simulink model "PI_park_filter_linearLoad"  (R2017b)
settings: Solver=ode23tb  StartTime=0.0  StopTime=.6  MaxStep=1e-4  RelTol=1e-3
undefined symbols (not defined in the file): D1, Delta
libraries: powerlib x42, powerlib_extras x9, powerlib_meascontrol x3, sdolib x1, peSinusoidalMeasurement x1
settings Model: Creator=HP  LastModifiedBy=HP

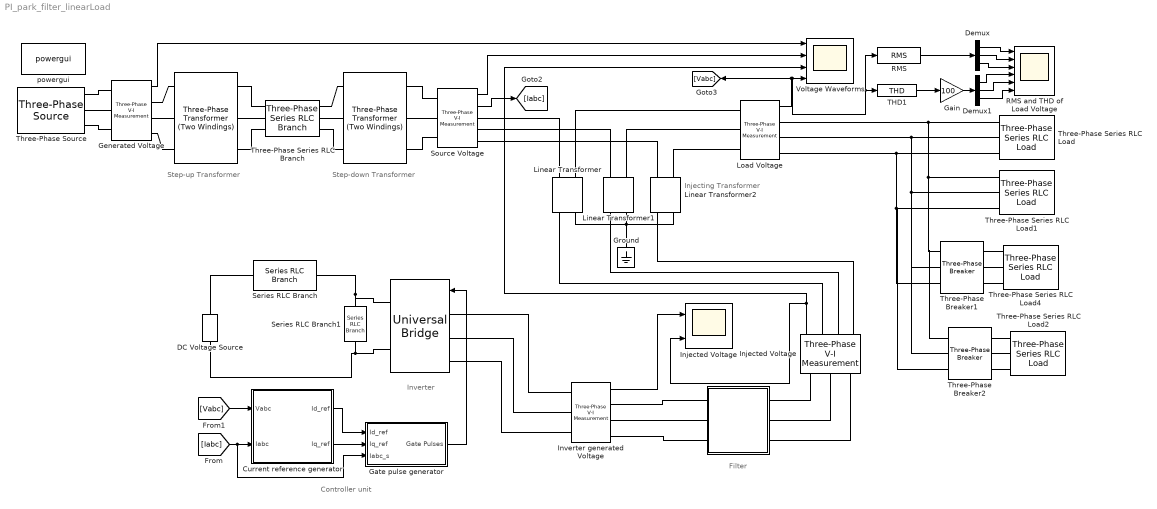
== system PI_park_filter_linearLoad ==
  note: Step-up Transformer
  note: Controller unit
  note: Injecting Transformer
  note: Step-down Transformer
  note: Inverter
  note: Filter
  " " : powerlib/Elements/Three-Phase Transformer (Two Windings)  Winding1Connection=Yg  Winding2Connection=Delta (D1)  CoreType=Three single-phase transformers  SetSaturation=off  Hysteresis=off  DataFile='hysteresis'  SetInitialFlux=off  Measurements=None  UNITS=pu  NominalPower=[ 70e6 , 50 ]  Winding1=[ 13e3 , 0.002 , 0.08 ]  Winding2=[ 115e3 , 0.002 , 0.08 ]  Rm=500  Lm=1400  L0=0.5  Saturation=[ 0,0 ; 0.0024,1.2 ; 1.0,1.52 ]  InitialFluxes=[ 0.8 , -0.8 , 0.7 ]  MoreParameters=off  BreakLoop=off  DataType=off  TransfoNumber=1
  " " : Subsystem
  "      " : powerlib/Elements/Three-Phase Transformer (Two Windings)  Winding1Connection=Delta (D1)  Winding2Connection=Yg  CoreType=Three single-phase transformers  SetSaturation=off  Hysteresis=off  DataFile='hysteresis'  SetInitialFlux=off  Measurements=None  UNITS=pu  NominalPower=[ 70e6 , 50 ]  Winding1=[ 115e3 , 0.002 , 0.08 ]  Winding2=[ 11e3 , 0.002 , 0.08 ]  Rm=500  Lm=800  L0=0.5  Saturation=[ 0,0 ; 0.0024,1.2 ; 1.0,1.52 ]  InitialFluxes=[ 0.8 , -0.8 , 0.7 ]  MoreParameters=off  BreakLoop=off  DataType=off  TransfoNumber=1
  "                                 " : powerlib/Power Electronics/Universal Bridge  Arms=3  SnubberResistance=1e5  SnubberCapacitance=inf  Device=IGBT / Diodes  Ron=1  Lon=0  ForwardVoltages="[  0  0  ]"  ForwardVoltage=0  GTOparameters=[ 10e-6 , 20e-6 ]  IGBTparameters=[ 1e-6 , 2e-6 ]  Measurements=None  Measurements_2=None  converterType=Rectifier
  Current reference generator : Subsystem
  "DC Voltage Source " : powerlib/Electrical Sources/DC Voltage Source  Amplitude=400  Measurements=None
  Demux : Demux  Outputs=3
  Demux1 : Demux  Outputs=3
  Gain : Gain  Gain=100
  "Gate pulse generator " : Subsystem
  Generated Voltage : powerlib/Measurements/Three-Phase V-I Measurement  VoltageMeasurement=phase-to-ground  SetLabelV=off  LabelV=Vabc  Vpu=off  VpuLL=off  CurrentMeasurement=no  SetLabelI=off  LabelI=Iabc  Ipu=off  Pbase=100e6  Vbase=11e3  OutputType=Complex  PhasorSimulation=off  PSBequivalent=0
  Ground : powerlib/Elements/Ground  LConnTagsString=a
  Injected Voltage : powerlib/Measurements/Three-Phase V-I Measurement  VoltageMeasurement=phase-to-ground  SetLabelV=off  LabelV=Vabc  Vpu=off  VpuLL=off  CurrentMeasurement=no  SetLabelI=off  LabelI=Iabc  Ipu=off  Pbase=100e6  Vbase=11e3  OutputType=Complex  PhasorSimulation=off  PSBequivalent=0
  "Injected Voltage " : Scope  NumInputPorts=2
  Inverter generated Voltage : powerlib/Measurements/Three-Phase V-I Measurement  VoltageMeasurement=phase-to-ground  SetLabelV=off  LabelV=Vabc  Vpu=off  VpuLL=off  CurrentMeasurement=no  SetLabelI=off  LabelI=Iabc  Ipu=off  Pbase=100e6  Vbase=11e3  OutputType=Complex  PhasorSimulation=off  PSBequivalent=0
  Linear Transformer : powerlib/Elements/Linear Transformer  UNITS=pu  NominalPower=[ 250e6 50 ]  winding1="[ 11e3  0.002  0.08 ]"  winding2="[ 22e3  0.002  0.08 ]"  ThreeWindings=off  winding3=[ 315e3 0.002 0.08 ]  RmLm=[ 500 750 ]  Measurements=None  DataType=off
  Linear Transformer1 : powerlib/Elements/Linear Transformer  UNITS=pu  NominalPower=[ 250e6 50 ]  winding1="[ 11e3  0.002  0.08 ]"  winding2="[ 22e3  0.002  0.08 ]"  ThreeWindings=off  winding3=[ 315e3 0.002 0.08 ]  RmLm=[ 500 750 ]  Measurements=None  DataType=off
  Linear Transformer2 : powerlib/Elements/Linear Transformer  UNITS=pu  NominalPower=[ 250e6 50 ]  winding1="[ 11e3  0.002  0.08 ]"  winding2="[ 22e3  0.002  0.08 ]"  ThreeWindings=off  winding3=[ 315e3 0.002 0.08 ]  RmLm=[ 500 750 ]  Measurements=None  DataType=off
  Load Voltage : powerlib/Measurements/Three-Phase V-I Measurement  VoltageMeasurement=phase-to-ground  SetLabelV=off  LabelV=Vabc  Vpu=off  VpuLL=off  CurrentMeasurement=no  SetLabelI=off  LabelI=Iabc  Ipu=off  Pbase=100e6  Vbase=11e3  OutputType=Complex  PhasorSimulation=off  PSBequivalent=0
  RMS : powerlib_meascontrol/Measurements/RMS  TrueRMS=on  Freq=50  RMSInit=120  Ts=0
  RMS and THD of Load Voltage : Scope  NumInputPorts=6
  Series RLC Branch : powerlib/Elements/Series RLC Branch  LConnTagsString=__new0  RConnTagsString=__new0  BranchType=R  Resistance=20  Inductance=0  SetiL0=off  InitialCurrent=0  Capacitance=0  Setx0=off  InitialVoltage=0  Measurements=None
  Series RLC Branch1 : powerlib/Elements/Series RLC Branch  LConnTagsString=__new0  RConnTagsString=__new0  BranchType=C  Resistance=10  Inductance=0  SetiL0=off  InitialCurrent=0  Capacitance=1e-3  Setx0=off  InitialVoltage=0  Measurements=None
  Source Voltage : powerlib/Measurements/Three-Phase V-I Measurement  VoltageMeasurement=phase-to-ground  SetLabelV=off  LabelV=Vabc  Vpu=off  VpuLL=off  CurrentMeasurement=yes  SetLabelI=off  LabelI=Iabc  Ipu=off  Pbase=100e6  Vbase=11e3  OutputType=Complex  PhasorSimulation=off  PSBequivalent=0
  THD1 : powerlib_meascontrol/Measurements/THD  Freq=50  Ts=0
  Three-Phase Series RLC Branch : powerlib/Elements/Three-Phase Series RLC Branch  LConnTagsString=A|B|C  RConnTagsString=A|B|C  BranchType=RL  Resistance=.1  Inductance=.5e-3  Capacitance=1e-6  Measurements=None
  Three-Phase Series RLC Load : powerlib/Elements/Three-Phase Series RLC Load  LConnTagsString=A|B|C  Configuration=Y (grounded)  NominalVoltage=11000  Vabc=[1e3 1e3 1e3]  Vabcp=[1e3 1e3 1e3]  NominalFrequency=50  UnbalancedPower=off  ActivePower=20e3  InductivePower=60e3  CapacitivePower=0  Pabc=[10e3 9e3 11e3]  QLabc=[100 90 110]  QCabc=[100 90 110]  Pabcp=[10e3 9e3 11e3]  QLabcp=[100 90 110]  QCabcp=[100 90 110]  Measurements=None  LoadType=constant Z
  Three-Phase Series RLC Load1 : powerlib/Elements/Three-Phase Series RLC Load  LConnTagsString=A|B|C  Configuration=Y (grounded)  NominalVoltage=11000  Vabc=[1e3 1e3 1e3]  Vabcp=[1e3 1e3 1e3]  NominalFrequency=50  UnbalancedPower=off  ActivePower=20e3  InductivePower=60e3  CapacitivePower=0  Pabc=[10e3 9e3 11e3]  QLabc=[100 90 110]  QCabc=[100 90 110]  Pabcp=[10e3 9e3 11e3]  QLabcp=[100 90 110]  QCabcp=[100 90 110]  Measurements=None  LoadType=constant Z
  Three-Phase Series RLC Load2 : powerlib/Elements/Three-Phase Series RLC Load  LConnTagsString=A|B|C  Configuration=Y (grounded)  NominalVoltage=11000  Vabc=[1e3 1e3 1e3]  Vabcp=[1e3 1e3 1e3]  NominalFrequency=50  UnbalancedPower=off  ActivePower=300e3  InductivePower=0  CapacitivePower=0  Pabc=[10e3 9e3 11e3]  QLabc=[100 90 110]  QCabc=[100 90 110]  Pabcp=[10e3 9e3 11e3]  QLabcp=[100 90 110]  QCabcp=[100 90 110]  Measurements=None  LoadType=constant Z
  Three-Phase Series RLC Load4 : powerlib/Elements/Three-Phase Series RLC Load  LConnTagsString=A|B|C  Configuration=Y (grounded)  NominalVoltage=11000  Vabc=[1e3 1e3 1e3]  Vabcp=[1e3 1e3 1e3]  NominalFrequency=50  UnbalancedPower=off  ActivePower=350e3  InductivePower=0  CapacitivePower=0  Pabc=[10e3 9e3 11e3]  QLabc=[100 90 110]  QCabc=[100 90 110]  Pabcp=[10e3 9e3 11e3]  QLabcp=[100 90 110]  QCabcp=[100 90 110]  Measurements=None  LoadType=constant Z
  Three-Phase Breaker1 : powerlib/Elements/Three-Phase Breaker  InitialState=open  SwitchA=on  SwitchB=on  SwitchC=on  SwitchTimes="[10/50  ]"  External=off  BreakerResistance=0.01  SnubberResistance=1e6  SnubberCapacitance=inf  Measurements=None
  Three-Phase Breaker2 : powerlib/Elements/Three-Phase Breaker  InitialState=open  SwitchA=on  SwitchB=on  SwitchC=on  SwitchTimes="[20/50  ]"  External=off  BreakerResistance=0.01  SnubberResistance=1e6  SnubberCapacitance=inf  Measurements=None
  Three-Phase Source : powerlib/Electrical Sources/Three-Phase Source  InternalConnection=Yg  VoltagePhases=off  Voltage=13e3  PhaseAngle=0  Voltage_phases=[25e3 25e3 25e3]/sqrt(3)  PhaseAngles_phases=[0 -120 +120]  Frequency=50  NonIdealSource=on  SpecifyImpedance=off  Resistance=0.2929  Inductance=16.58e-3  ShortCircuitLevel=100e6  BaseVoltage=13e3  XRratio=7  BusType=swing  Pref=10e3  Qref=0  Prefabc=[10e3, 10e3, 10e3]  Qrefabc=[0, 0, 0]  Qmin=-inf  Qmax=inf
  "Voltage Waveforms " : Scope  NumInputPorts=4
  powergui : powerlib/powergui  Priority=1  SimulationMode=Discrete  SampleTime=50e-6  frequency=60  Iterations=50  frequencyindice=50  Pbase=100e6  ErrMax=1e-4  UnitsV=kV  UnitsW=MW  buscounter=0  FunctionMessages=off  echomessages=off  EnableUseOfTLC=off  CurrentSourceSwitches=off  DisableSnubberDevices=off  DisableRonSwitches=off  DisableVfSwitches=off  DisplayEquations=off  SolverType=Tustin/Backward Euler (TBE)  Interpol=off  ExternalGateDelay=off  methode=off  Ts=100  x0status=blocks  SPID=on  SwTol=0  HookPort=off  RestoreLinks=warning  ResistiveCurrentMeasurement=off  Frange=[0:2:500]  Ylog=off  Xlog=on  ShowGrid=off  save=off  variable=ZData  structure=WAVEFORMS_PI_PARK_Linear  ZoomFFT=off  StartTime=0.  cycles=30  DisplayStyle=1  fundamental=50  FreqAxis=off  MaxFrequency=1000  frequencyindicesteady=1  RmsSteady=1  display=off
  wires:
  [Vabc] -> Current reference generator/1(Vabc)
  [Iabc] -> "Gate pulse generator "/3(Iabc_s), Current reference generator/2(Iabc)
  Current reference generator/1(Id_ref) -> "Gate pulse generator "/1(Id_ref)
  Current reference generator/2(Iq_ref) -> "Gate pulse generator "/2(Iq_ref)
  "Gate pulse generator "/1("Gate Pulses ") -> "                                 "/1
  Source Voltage/2 -> [Iabc]
  Load Voltage/1 -> RMS/1, THD1/1, "Voltage Waveforms "/4, [Vabc]
  Generated Voltage/1 -> "Voltage Waveforms "/1
  Source Voltage/1 -> "Voltage Waveforms "/2
  Injected Voltage/1 -> "Injected Voltage "/2, "Voltage Waveforms "/3
  Inverter generated Voltage/1 -> "Injected Voltage "/1
  Demux/1 -> RMS and THD of Load Voltage/1
  Demux/2 -> RMS and THD of Load Voltage/2
  Demux/3 -> RMS and THD of Load Voltage/3
  Demux1/2 -> RMS and THD of Load Voltage/5
  Demux1/1 -> RMS and THD of Load Voltage/4
  Demux1/3 -> RMS and THD of Load Voltage/6
  THD1/1 -> Gain/1
  Gain/1 -> Demux1/1
  RMS/1 -> Demux/1
  connections:
  "DC Voltage Source "/RConn1 -- Series RLC Branch/LConn1
  Series RLC Branch1/LConn1 -- "                                 "/RConn1 -- Series RLC Branch/RConn1
  "DC Voltage Source "/LConn1 -- "                                 "/RConn2 -- Series RLC Branch1/RConn1
  Three-Phase Series RLC Load1/LConn3 -- Three-Phase Breaker2/LConn3 -- Three-Phase Breaker1/LConn3 -- Three-Phase Series RLC Load/LConn3 -- Load Voltage/RConn3
  Three-Phase Series RLC Load1/LConn1 -- Three-Phase Breaker2/LConn1 -- Three-Phase Breaker1/LConn1 -- Three-Phase Series RLC Load/LConn1 -- Load Voltage/RConn1
  Three-Phase Series RLC Load1/LConn2 -- Three-Phase Breaker2/LConn2 -- Three-Phase Breaker1/LConn2 -- Load Voltage/RConn2 -- Three-Phase Series RLC Load/LConn2
  Linear Transformer2/LConn1 -- Load Voltage/LConn3
  " "/LConn2 -- Generated Voltage/RConn2
  Three-Phase Series RLC Branch/LConn1 -- " "/RConn1
  Generated Voltage/RConn1 -- " "/LConn1
  "      "/RConn3 -- Source Voltage/LConn3
  Three-Phase Source/RConn3 -- Generated Voltage/LConn3
  " "/LConn3 -- Generated Voltage/RConn3
  Source Voltage/LConn1 -- "      "/RConn1
  Three-Phase Source/RConn1 -- Generated Voltage/LConn1
  Three-Phase Series RLC Branch/LConn2 -- " "/RConn2
  Generated Voltage/LConn2 -- Three-Phase Source/RConn2
  Linear Transformer/LConn1 -- Load Voltage/LConn1
  Source Voltage/RConn1 -- Linear Transformer/LConn2
  Load Voltage/LConn2 -- Linear Transformer1/LConn1
  Source Voltage/RConn3 -- Linear Transformer2/LConn2
  Source Voltage/LConn2 -- "      "/RConn2
  Three-Phase Series RLC Branch/RConn1 -- "      "/LConn1
  Three-Phase Series RLC Branch/RConn3 -- "      "/LConn3
  Three-Phase Series RLC Branch/RConn2 -- "      "/LConn2
  Three-Phase Series RLC Branch/LConn3 -- " "/RConn3
  Source Voltage/RConn2 -- Linear Transformer1/LConn2
  Linear Transformer/RConn1 -- Ground/LConn1 -- Linear Transformer1/RConn1 -- Linear Transformer2/RConn1
  Injected Voltage/RConn1 -- Linear Transformer/RConn2
  Injected Voltage/RConn2 -- Linear Transformer1/RConn2
  Injected Voltage/RConn3 -- Linear Transformer2/RConn2
  Inverter generated Voltage/LConn1 -- "                                 "/LConn1
  Inverter generated Voltage/LConn2 -- "                                 "/LConn2
  Inverter generated Voltage/LConn3 -- "                                 "/LConn3
  " "/RConn1 -- Injected Voltage/LConn1
  " "/RConn2 -- Injected Voltage/LConn2
  " "/RConn3 -- Injected Voltage/LConn3
  Inverter generated Voltage/RConn1 -- " "/LConn1
  Inverter generated Voltage/RConn2 -- " "/LConn2
  Inverter generated Voltage/RConn3 -- " "/LConn3
  Three-Phase Series RLC Load4/LConn3 -- Three-Phase Breaker1/RConn3
  Three-Phase Series RLC Load4/LConn2 -- Three-Phase Breaker1/RConn2
  Three-Phase Series RLC Load4/LConn1 -- Three-Phase Breaker1/RConn1
  Three-Phase Series RLC Load2/LConn1 -- Three-Phase Breaker2/RConn1
  Three-Phase Series RLC Load2/LConn2 -- Three-Phase Breaker2/RConn2
  Three-Phase Series RLC Load2/LConn3 -- Three-Phase Breaker2/RConn3

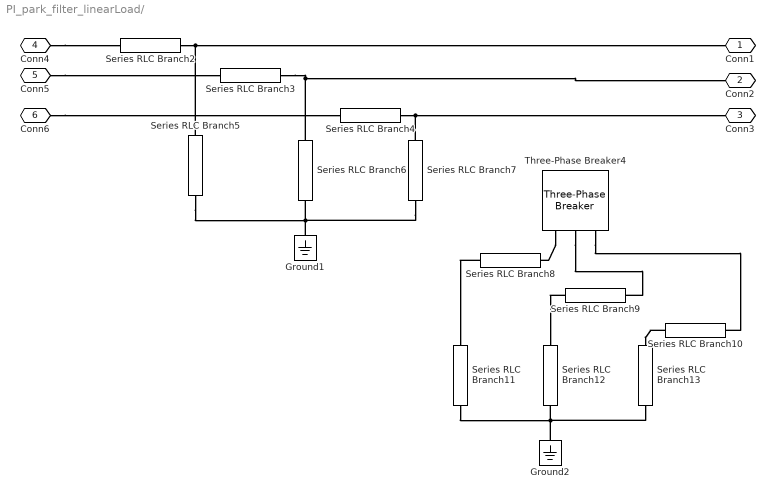
== system PI_park_filter_linearLoad/  ==
  Ground1 : powerlib/Elements/Ground  LConnTagsString=a
  Ground2 : powerlib/Elements/Ground  LConnTagsString=a
  Series RLC Branch10 : powerlib/Elements/Series RLC Branch  LConnTagsString=__new0  RConnTagsString=__new0  BranchType=RL  Resistance=20  Inductance=7e-3  SetiL0=off  InitialCurrent=0  Capacitance=1e-6  Setx0=off  InitialVoltage=0  Measurements=None
  Series RLC Branch{5..7,11..13} (6 alike) : powerlib/Elements/Series RLC Branch  LConnTagsString=__new0  RConnTagsString=__new0  BranchType=RC  Resistance=5  Inductance=50e-6  SetiL0=off  InitialCurrent=0  Capacitance=50e-6  Setx0=off  InitialVoltage=0  Measurements=None
  Series RLC Branch2 : powerlib/Elements/Series RLC Branch  LConnTagsString=__new0  RConnTagsString=__new0  BranchType=RL  Resistance=50  Inductance=7e-3  SetiL0=off  InitialCurrent=0  Capacitance=1e-6  Setx0=off  InitialVoltage=0  Measurements=None
  Series RLC Branch3 : powerlib/Elements/Series RLC Branch  LConnTagsString=__new0  RConnTagsString=__new0  BranchType=RL  Resistance=50  Inductance=7e-3  SetiL0=off  InitialCurrent=0  Capacitance=1e-6  Setx0=off  InitialVoltage=0  Measurements=None
  Series RLC Branch4 : powerlib/Elements/Series RLC Branch  LConnTagsString=__new0  RConnTagsString=__new0  BranchType=RL  Resistance=50  Inductance=7e-3  SetiL0=off  InitialCurrent=0  Capacitance=1e-6  Setx0=off  InitialVoltage=0  Measurements=None
  Series RLC Branch8 : powerlib/Elements/Series RLC Branch  LConnTagsString=__new0  RConnTagsString=__new0  BranchType=RL  Resistance=20  Inductance=7e-3  SetiL0=off  InitialCurrent=0  Capacitance=1e-6  Setx0=off  InitialVoltage=0  Measurements=None
  Series RLC Branch9 : powerlib/Elements/Series RLC Branch  LConnTagsString=__new0  RConnTagsString=__new0  BranchType=RL  Resistance=20  Inductance=7e-3  SetiL0=off  InitialCurrent=0  Capacitance=1e-6  Setx0=off  InitialVoltage=0  Measurements=None
  Three-Phase Breaker4 : powerlib/Elements/Three-Phase Breaker  InitialState=open  SwitchA=on  SwitchB=on  SwitchC=on  SwitchTimes="[20/50  ]"  External=off  BreakerResistance=0.01  SnubberResistance=1e6  SnubberCapacitance=inf  Measurements=None
  Conn1 : PMIOPort  Port=1  Side=Right
  Conn2 : PMIOPort  Port=2  Side=Right
  Conn3 : PMIOPort  Port=3  Side=Right
  Conn4 : PMIOPort  Port=4  Side=Left
  Conn5 : PMIOPort  Port=5  Side=Left
  Conn6 : PMIOPort  Port=6  Side=Left
  connections:
  Series RLC Branch8/RConn1 -- Series RLC Branch11/LConn1
  Series RLC Branch10/RConn1 -- Series RLC Branch13/LConn1
  Series RLC Branch5/RConn1 -- Ground1/LConn1 -- Series RLC Branch7/RConn1 -- Series RLC Branch6/RConn1
  Series RLC Branch4/RConn1 -- Conn3/RConn1 -- Series RLC Branch7/LConn1
  Series RLC Branch11/RConn1 -- Series RLC Branch13/RConn1 -- Ground2/LConn1 -- Series RLC Branch12/RConn1
  Three-Phase Breaker4/RConn2 -- Series RLC Branch9/LConn1
  Conn4/RConn1 -- Series RLC Branch2/LConn1
  Conn5/RConn1 -- Series RLC Branch3/LConn1
  Three-Phase Breaker4/RConn1 -- Series RLC Branch8/LConn1
  Series RLC Branch2/RConn1 -- Conn1/RConn1 -- Series RLC Branch5/LConn1
  Three-Phase Breaker4/RConn3 -- Series RLC Branch10/LConn1
  Conn6/RConn1 -- Series RLC Branch4/LConn1
  Series RLC Branch3/RConn1 -- Series RLC Branch6/LConn1 -- Conn2/RConn1
  Series RLC Branch9/RConn1 -- Series RLC Branch12/LConn1

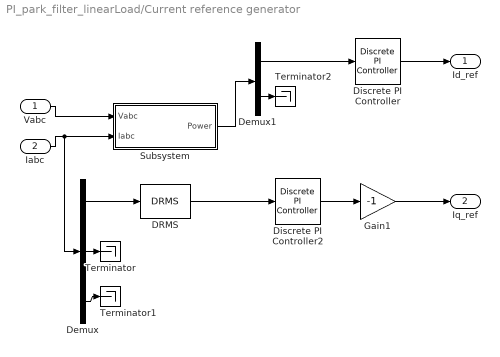
== system PI_park_filter_linearLoad/Current reference generator ==
  Vabc : Inport
  Iabc : Inport  Port=2
  DRMS : sdolib/RMS Blocks/DRMS  Ts=2e-6
      settings: SourceProductName=Simulink Design Optimization  SourceProductBaseCode=SO
  Demux : Demux  Outputs=3
  Demux1 : Demux  Outputs=2
  Discrete PI Controller : powerlib_extras/Discrete  Control Blocks/Discrete PI Controller  Kp=0.4  Ki=3000  Par_Limits=[1e6 -1e6]  Init=0  Ts=-1
  Discrete PI Controller2 : powerlib_extras/Discrete  Control Blocks/Discrete PI Controller  Kp=200  Ki=3800  Par_Limits=[1e6 -1e6]  Init=0  Ts=-1
  Gain1 : Gain  Gain=-1
  Subsystem : Subsystem
  Terminator : Terminator
  Terminator1 : Terminator
  Terminator2 : Terminator
  Id_ref : Outport
  Iq_ref : Outport  Port=2
  wires:
  DRMS/1 -> Discrete PI Controller2/1
  Discrete PI Controller/1 -> Id_ref/1
  Demux1/1 -> Discrete PI Controller/1
  Vabc/1 -> Subsystem/1(Vabc)
  Iabc/1 -> Demux/1, Subsystem/2(Iabc)
  Gain1/1 -> Iq_ref/1
  Discrete PI Controller2/1 -> Gain1/1
  Subsystem/1(Power) -> Demux1/1
  Demux1/2 -> Terminator2/1
  Demux/2 -> Terminator/1
  Demux/3 -> Terminator1/1
  Demux/1 -> DRMS/1

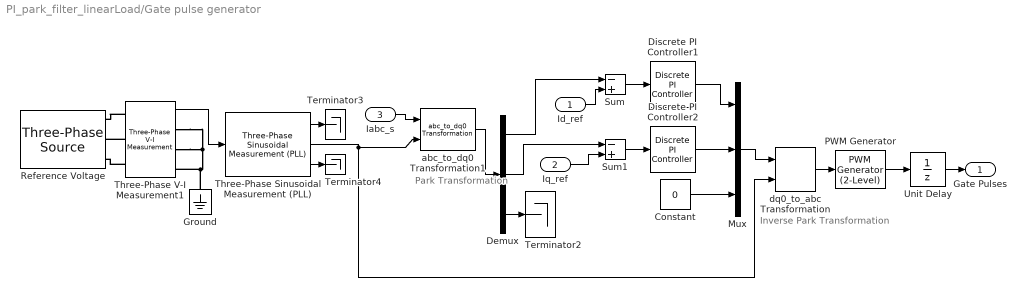
== system PI_park_filter_linearLoad/Gate pulse generator  ==
  note: Park
      | Transformation
  note: Inverse
      | Park
      | Transformation
  Id_ref : Inport
  Iq_ref : Inport  Port=2
  Iabc_s : Inport  Port=3
  Constant : Constant  Value=0  SampleTime=-1
  Demux : Demux  Outputs=3
  Discrete PI Controller1 : powerlib_extras/Discrete  Control Blocks/Discrete PI Controller  Kp=4  Ki=2000  Par_Limits=[1e6 -1e6]  Init=0  Ts=-1
  Discrete PI Controller2 : powerlib_extras/Discrete  Control Blocks/Discrete PI Controller  Kp=4  Ki=2000  Par_Limits=[1e6 -1e6]  Init=0  Ts=-1
  Ground : powerlib/Elements/Ground  LConnTagsString=a
  Mux : Mux  Inputs=3
  "PWM Generator " : powerlib_meascontrol/Pulse & Signal Generators/PWM Generator (2-Level)  ModulatorType=Three-phase bridge (6 pulses)  ModulatorMode=Unsynchronized  Fc=10000  Pc=90  nF=27  MinMax="[ -1  1 ]"  SamplingTechnique=Natural  ModulatingSignals=off  m=0.8  Freq=60  Phase=0  Ts=2  ShowCarrierOutport=off
      settings: SourceProductName=Simscape Power Systems
  Reference Voltage : powerlib/Electrical Sources/Three-Phase Source  InternalConnection=Yg  VoltagePhases=off  Voltage=11e3  PhaseAngle=0  Voltage_phases=[25e3 25e3 25e3]/sqrt(3)  PhaseAngles_phases=[0 -120 +120]  Frequency=50  NonIdealSource=on  SpecifyImpedance=off  Resistance=0.8929  Inductance=16.58e-3  ShortCircuitLevel=100e6  BaseVoltage=11e3  XRratio=7  BusType=swing  Pref=10e3  Qref=0  Prefabc=[10e3, 10e3, 10e3]  Qrefabc=[0, 0, 0]  Qmin=-inf  Qmax=inf
  Sum : Sum  Inputs=-+
  Sum1 : Sum  Inputs=-+
  Terminator2 : Terminator
  Terminator3 : Terminator
  Terminator4 : Terminator
  Three-Phase V-I Measurement1 : powerlib/Measurements/Three-Phase V-I Measurement  VoltageMeasurement=phase-to-ground  SetLabelV=off  LabelV=Vabc  Vpu=off  VpuLL=off  CurrentMeasurement=no  SetLabelI=off  LabelI=Iabc  Ipu=off  Pbase=100e6  Vbase=500e3  OutputType=Complex  PhasorSimulation=off  PSBequivalent=0
  Three-Phase Sinusoidal Measurement (PLL) : peSinusoidalMeasurement/Three-Phase Sinusoidal Measurement (PLL)  Kp_LF=200  Ki_LF=2000  F0=50  Theta0=0  Ts=-1
  Unit Delay : UnitDelay  SampleTime=-1
  abc_to_dq0 Transformation1 : powerlib_extras/Measurements/abc_to_dq0 Transformation
  dq0_to_abc Transformation : powerlib_extras/Measurements/dq0_to_abc Transformation
  "Gate Pulses " : Outport
  wires:
  Three-Phase Sinusoidal Measurement (PLL)/2 -> dq0_to_abc Transformation/2, abc_to_dq0 Transformation1/2
  Iabc_s/1 -> abc_to_dq0 Transformation1/1
  abc_to_dq0 Transformation1/1 -> Demux/1
  Demux/1 -> Sum/1
  Id_ref/1 -> Sum/2
  Demux/2 -> Sum1/1
  Iq_ref/1 -> Sum1/2
  Sum/1 -> Discrete PI Controller1/1
  Sum1/1 -> Discrete PI Controller2/1
  Discrete PI Controller1/1 -> Mux/1
  Discrete PI Controller2/1 -> Mux/2
  Constant/1 -> Mux/3
  Mux/1 -> dq0_to_abc Transformation/1
  dq0_to_abc Transformation/1 -> "PWM Generator "/1
  "PWM Generator "/1 -> Unit Delay/1
  Unit Delay/1 -> "Gate Pulses "/1
  Demux/3 -> Terminator2/1
  Three-Phase Sinusoidal Measurement (PLL)/1 -> Terminator3/1
  Three-Phase Sinusoidal Measurement (PLL)/3 -> Terminator4/1
  Three-Phase V-I Measurement1/1 -> Three-Phase Sinusoidal Measurement (PLL)/1
  connections:
  Three-Phase V-I Measurement1/LConn1 -- Reference Voltage/RConn1
  Three-Phase V-I Measurement1/LConn2 -- Reference Voltage/RConn2
  Three-Phase V-I Measurement1/LConn3 -- Reference Voltage/RConn3
  Three-Phase V-I Measurement1/RConn1 -- Three-Phase V-I Measurement1/RConn2 -- Three-Phase V-I Measurement1/RConn3 -- Ground/LConn1

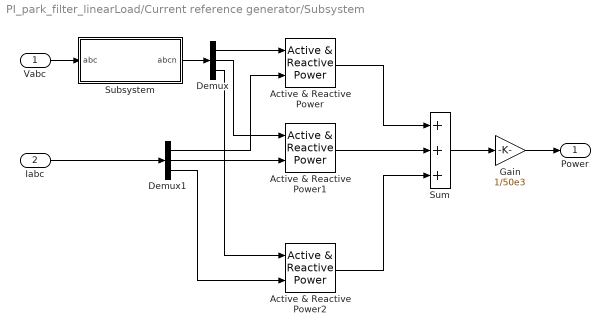
== system PI_park_filter_linearLoad/Current reference generator/Subsystem ==
  Vabc : Inport
  Iabc : Inport  Port=2
  Active & Reactive Power : powerlib_extras/Measurements/Active & Reactive Power  f1=50
      link override I_Fundamental: f1=f1
      link override V_Fundamental: f1=f1
  Active & Reactive Power1 : powerlib_extras/Measurements/Active & Reactive Power  f1=50
  Active & Reactive Power2 : powerlib_extras/Measurements/Active & Reactive Power  f1=50
  Demux : Demux  Outputs=3
  Demux1 : Demux  Outputs=3
  Gain : Gain  Gain=1/50e3
  Subsystem : Subsystem
  Sum : Sum  Inputs=3
  Power : Outport
  wires:
  Vabc/1 -> Subsystem/1(abc)
  Subsystem/1(abcn) -> Demux/1
  Demux/1 -> Active & Reactive Power/1
  Iabc/1 -> Demux1/1
  Demux1/1 -> Active & Reactive Power/2
  Demux1/2 -> Active & Reactive Power1/2
  Demux/2 -> Active & Reactive Power1/1
  Demux/3 -> Active & Reactive Power2/1
  Demux1/3 -> Active & Reactive Power2/2
  Active & Reactive Power1/1 -> Sum/2
  Active & Reactive Power/1 -> Sum/1
  Active & Reactive Power2/1 -> Sum/3
  Sum/1 -> Gain/1
  Gain/1 -> Power/1

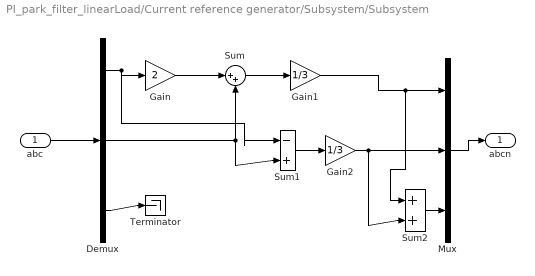
== system PI_park_filter_linearLoad/Current reference generator/Subsystem/Subsystem ==
  abc : Inport
  Demux : Demux  Outputs=3
  Gain : Gain  Gain=2
  Gain1 : Gain  Gain=1/3
  Gain2 : Gain  Gain=1/3
  Mux : Mux  Inputs=3
  Sum : Sum  Inputs=|++
  Sum1 : Sum  Inputs=|-+
  Sum2 : Sum  Inputs=|++
  Terminator : Terminator
  abcn : Outport
  wires:
  abc/1 -> Demux/1
  Gain/1 -> Sum/1
  Demux/2 -> Sum1/2, Sum/2
  Sum/1 -> Gain1/1
  Mux/1 -> abcn/1
  Gain1/1 -> Sum2/1, Mux/1
  Demux/1 -> Sum1/1, Gain/1
  Demux/3 -> Terminator/1
  Sum1/1 -> Gain2/1
  Gain2/1 -> Sum2/2, Mux/2
  Sum2/1 -> Mux/3
